simulink model "v14_registers"  (R2019b)
settings: Solver=FixedStepAuto  StartTime=0.0  StopTime=inf  FixedStep=1  MaxStep=1  RelTol=1e-3
libraries: simulink x4
settings Model: Creator=MARAT  LastModifiedBy=Marat
settings SFSimCC: CustomCodeUndefinedFunction=UseInterfaceOnly

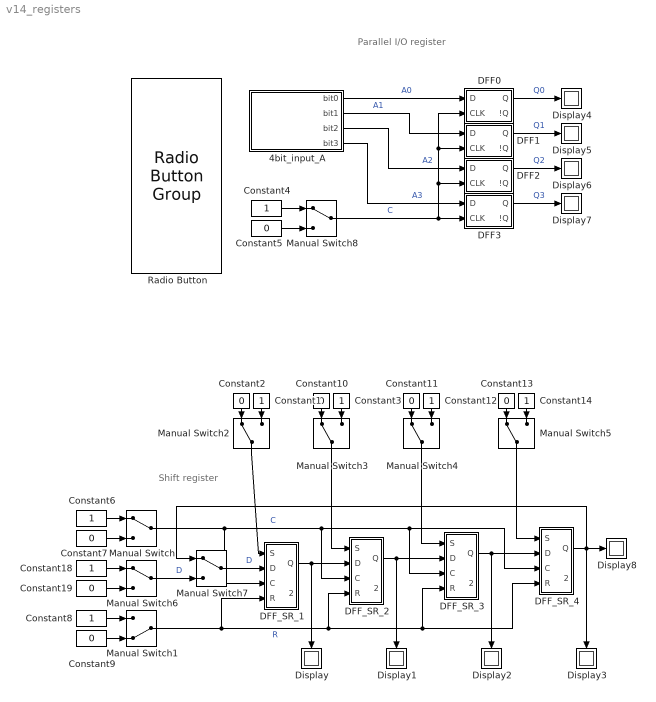
== system v14_registers ==
  note: Parallel I/O register
  note: Shift register
  4bit_input_A : Subsystem
      mask Display: image('images\sansA.png'); % Use "Edit Image" on toolstrip to change.
  Constant{1,3..4,6,8,12,14,18} (8 alike) : Constant  OutDataTypeStr=boolean
  Constant{2,5,7,9..11,13,19} (8 alike) : Constant  Value=0  OutDataTypeStr=boolean
  DFF0 : Subsystem
  DFF1 : Subsystem
  DFF2 : Subsystem
  DFF3 : Subsystem
  DFF_SR_1 : Subsystem
  DFF_SR_2 : Subsystem
  DFF_SR_3 : Subsystem
  DFF_SR_4 : Subsystem
  Display{,1..8} (9 alike) : Display
  Manual Switch{,2..8} (8 alike) : ManualSwitch
  Manual Switch1 : ManualSwitch  CurrentSetting=0
  Radio Button : RadioButtonGroup  SelectedLabel=0
      settings: Values={{'0', '1', '2', '3', '4', '5', '6', '7', '8', '9', '10', '11', '12', '13', '14', '15'}, [0 1 2 3 4 5 6 7 8 9 10 11 12 13 14 15]}
  wires:
  4bit_input_A/1(bit0) -> DFF0/1(D)  "A0"
  4bit_input_A/2(bit1) -> DFF1/1(D)  "A1"
  4bit_input_A/3(bit2) -> DFF2/1(D)  "A2"
  4bit_input_A/4(bit3) -> DFF3/1(D)  "A3"
  Constant5/1 -> Manual Switch8/2
  Constant4/1 -> Manual Switch8/1
  Manual Switch8/1 -> DFF3/2(CLK), DFF2/2(CLK), DFF1/2(CLK), DFF0/2(CLK)  "C"
  Manual Switch1/1 -> DFF_SR_4/4(R), DFF_SR_3/4(R), DFF_SR_2/4(R), DFF_SR_1/4(R)  "R"
  DFF_SR_1/1(Q) -> Display/1, DFF_SR_2/2(D)
  DFF_SR_2/1(Q) -> DFF_SR_3/2(D), Display1/1
  DFF_SR_3/1(Q) -> DFF_SR_4/2(D), Display2/1
  Constant6/1 -> Manual Switch/1
  Constant7/1 -> Manual Switch/2
  Manual Switch/1 -> DFF_SR_4/3(C), DFF_SR_3/3(C), DFF_SR_2/3(C), DFF_SR_1/3(C)  "C"
  DFF_SR_4/1(Q) -> Manual Switch7/1, Display8/1, Display3/1
  Constant9/1 -> Manual Switch1/2
  Constant8/1 -> Manual Switch1/1
  DFF0/1(Q) -> Display4/1  "Q0"
  DFF1/1(Q) -> Display5/1  "Q1"
  DFF2/1(Q) -> Display6/1  "Q2"
  DFF3/1(Q) -> Display7/1  "Q3"
  Constant19/1 -> Manual Switch6/2
  Constant18/1 -> Manual Switch6/1
  Manual Switch7/1 -> DFF_SR_1/2(D)  "D"
  Manual Switch6/1 -> Manual Switch7/2  "D"
  Manual Switch4/1 -> DFF_SR_3/1(S)
  Manual Switch5/1 -> DFF_SR_4/1(S)
  Manual Switch3/1 -> DFF_SR_2/1(S)
  Manual Switch2/1 -> DFF_SR_1/1(S)
  Constant1/1 -> Manual Switch2/2
  Constant2/1 -> Manual Switch2/1
  Constant3/1 -> Manual Switch3/2
  Constant12/1 -> Manual Switch4/2
  Constant14/1 -> Manual Switch5/2
  Constant13/1 -> Manual Switch5/1
  Constant11/1 -> Manual Switch4/1
  Constant10/1 -> Manual Switch3/1

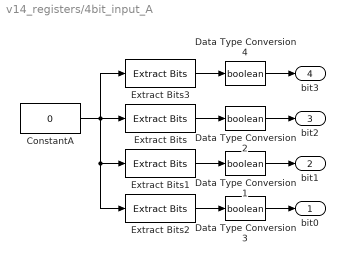
== system v14_registers/4bit_input_A ==
  ConstantA : Constant  Value=0  OutMin=0  OutMax=15  OutDataTypeStr=uint8
  Data Type Conversion{1..4} (4 alike) : DataTypeConversion  OutDataTypeStr=boolean
  Extract Bits : simulink/Logic and Bit Operations/Extract Bits  bitsToExtract=Range of bits  numBits=8  bitIdxRange=2  outScalingMode=Treat bit field as an integer
      settings: SourceProductName=Simulink
  Extract Bits1 : simulink/Logic and Bit Operations/Extract Bits  bitsToExtract=Range of bits  numBits=8  bitIdxRange=1  outScalingMode=Treat bit field as an integer
      settings: SourceProductName=Simulink
  Extract Bits2 : simulink/Logic and Bit Operations/Extract Bits  bitsToExtract=Range of bits  numBits=8  bitIdxRange=0  outScalingMode=Treat bit field as an integer
      settings: SourceProductName=Simulink
  Extract Bits3 : simulink/Logic and Bit Operations/Extract Bits  bitsToExtract=Range of bits  numBits=8  bitIdxRange=3  outScalingMode=Treat bit field as an integer
      settings: SourceProductName=Simulink
  bit0 : Outport
  bit1 : Outport  Port=2
  bit2 : Outport  Port=3
  bit3 : Outport  Port=4
  wires:
  ConstantA/1 -> Extract Bits3/1, Extract Bits2/1, Extract Bits1/1, Extract Bits/1
  Extract Bits/1 -> Data Type Conversion2/1
  Extract Bits1/1 -> Data Type Conversion1/1
  Extract Bits2/1 -> Data Type Conversion3/1
  Data Type Conversion2/1 -> bit2/1
  Data Type Conversion1/1 -> bit1/1
  Data Type Conversion3/1 -> bit0/1
  Data Type Conversion4/1 -> bit3/1
  Extract Bits3/1 -> Data Type Conversion4/1

== system v14_registers/DFF0 ==
  D : Inport
  CLK : Inport  Port=2
  Subsystem : Subsystem
  Q : Outport  InitialOutput=0  VectorParamsAs1DForOutWhenUnconnected=off
  !Q : Outport  Port=2  InitialOutput=1  VectorParamsAs1DForOutWhenUnconnected=off
  wires:
  Subsystem/2(!Q) -> !Q/1
  Subsystem/1(Q) -> Q/1
  D/1 -> Subsystem/1(D)
  CLK/1 -> Subsystem/Trigger

== system v14_registers/DFF1 ==
  D : Inport
  CLK : Inport  Port=2
  Subsystem : Subsystem
  Q : Outport  InitialOutput=0  VectorParamsAs1DForOutWhenUnconnected=off
  !Q : Outport  Port=2  InitialOutput=1  VectorParamsAs1DForOutWhenUnconnected=off
  wires:
  CLK/1 -> Subsystem/Trigger
  D/1 -> Subsystem/1(D)
  Subsystem/1(Q) -> Q/1
  Subsystem/2(!Q) -> !Q/1

== system v14_registers/DFF2 ==
  D : Inport
  CLK : Inport  Port=2
  Subsystem : Subsystem
  Q : Outport  InitialOutput=0  VectorParamsAs1DForOutWhenUnconnected=off
  !Q : Outport  Port=2  InitialOutput=1  VectorParamsAs1DForOutWhenUnconnected=off
  wires:
  Subsystem/2(!Q) -> !Q/1
  Subsystem/1(Q) -> Q/1
  D/1 -> Subsystem/1(D)
  CLK/1 -> Subsystem/Trigger

== system v14_registers/DFF3 ==
  D : Inport
  CLK : Inport  Port=2
  Subsystem : Subsystem
  Q : Outport  InitialOutput=0  VectorParamsAs1DForOutWhenUnconnected=off
  !Q : Outport  Port=2  InitialOutput=1  VectorParamsAs1DForOutWhenUnconnected=off
  wires:
  CLK/1 -> Subsystem/Trigger
  D/1 -> Subsystem/1(D)
  Subsystem/1(Q) -> Q/1
  Subsystem/2(!Q) -> !Q/1

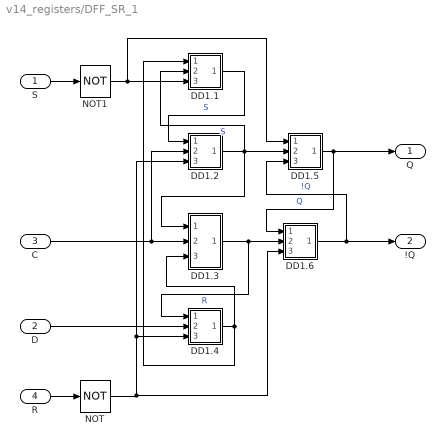
== system v14_registers/DFF_SR_1 ==
  S : Inport
  D : Inport  Port=2
  C : Inport  Port=3
  R : Inport  Port=4
  DD1.1 : Subsystem
      mask Display: disp('&~');
  DD1.2 : Subsystem
      mask Display: disp('&~');
  DD1.3 : Subsystem
      mask Display: disp('&~');
  DD1.4 : Subsystem
      mask Display: disp('&~');
  DD1.5 : Subsystem
      mask Display: disp('&~');
  DD1.6 : Subsystem
      mask Display: disp('&~');
  NOT : Logic  Operator=NOT  IconShape=distinctive  AllPortsSameDT=off  OutDataTypeStr=boolean
  NOT1 : Logic  Operator=NOT  IconShape=distinctive  AllPortsSameDT=off  OutDataTypeStr=boolean
  Q : Outport
  !Q : Outport  Port=2
  wires:
  DD1.5/1(Out1) -> Q/1, DD1.6/1(In1)  "Q"
  R/1 -> NOT/1
  DD1.4/1(Out1) -> DD1.1/1(In1), DD1.3/3(In3)
  C/1 -> DD1.2/2(In2), DD1.3/2(In2)
  S/1 -> NOT1/1
  DD1.3/1(Out1) -> DD1.6/2(In2), DD1.4/1(In1)  "R"
  DD1.1/1(Out1) -> DD1.2/1(In1)  "S"
  DD1.6/1(Out1) -> !Q/1, DD1.5/3(In3)  "!Q"
  D/1 -> DD1.4/2(In2)
  DD1.2/1(Out1) -> DD1.3/1(In1), DD1.5/2(In2), DD1.1/2(In2)  "S"
  NOT/1 -> DD1.6/3(In3), DD1.4/3(In3), DD1.2/3(In3)
  NOT1/1 -> DD1.5/1(In1), DD1.1/3(In3)

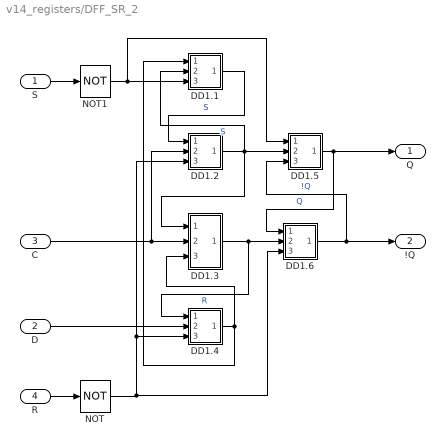
== system v14_registers/DFF_SR_2 ==
  S : Inport
  D : Inport  Port=2
  C : Inport  Port=3
  R : Inport  Port=4
  DD1.1 : Subsystem
      mask Display: disp('&~');
  DD1.2 : Subsystem
      mask Display: disp('&~');
  DD1.3 : Subsystem
      mask Display: disp('&~');
  DD1.4 : Subsystem
      mask Display: disp('&~');
  DD1.5 : Subsystem
      mask Display: disp('&~');
  DD1.6 : Subsystem
      mask Display: disp('&~');
  NOT : Logic  Operator=NOT  IconShape=distinctive  AllPortsSameDT=off  OutDataTypeStr=boolean
  NOT1 : Logic  Operator=NOT  IconShape=distinctive  AllPortsSameDT=off  OutDataTypeStr=boolean
  Q : Outport
  !Q : Outport  Port=2
  wires:
  NOT1/1 -> DD1.1/3(In3), DD1.5/1(In1)
  NOT/1 -> DD1.2/3(In3), DD1.4/3(In3), DD1.6/3(In3)
  DD1.2/1(Out1) -> DD1.1/2(In2), DD1.5/2(In2), DD1.3/1(In1)  "S"
  D/1 -> DD1.4/2(In2)
  DD1.6/1(Out1) -> DD1.5/3(In3), !Q/1  "!Q"
  DD1.1/1(Out1) -> DD1.2/1(In1)  "S"
  DD1.3/1(Out1) -> DD1.4/1(In1), DD1.6/2(In2)  "R"
  S/1 -> NOT1/1
  C/1 -> DD1.3/2(In2), DD1.2/2(In2)
  DD1.4/1(Out1) -> DD1.3/3(In3), DD1.1/1(In1)
  R/1 -> NOT/1
  DD1.5/1(Out1) -> DD1.6/1(In1), Q/1  "Q"

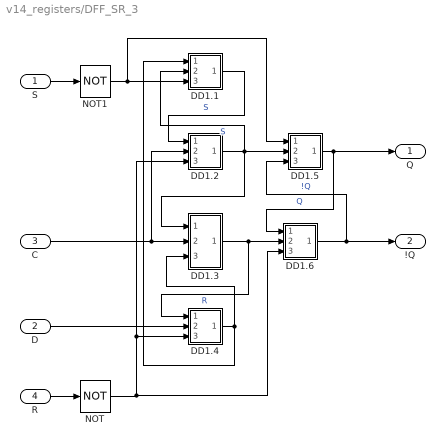
== system v14_registers/DFF_SR_3 ==
  S : Inport
  D : Inport  Port=2
  C : Inport  Port=3
  R : Inport  Port=4
  DD1.1 : Subsystem
      mask Display: disp('&~');
  DD1.2 : Subsystem
      mask Display: disp('&~');
  DD1.3 : Subsystem
      mask Display: disp('&~');
  DD1.4 : Subsystem
      mask Display: disp('&~');
  DD1.5 : Subsystem
      mask Display: disp('&~');
  DD1.6 : Subsystem
      mask Display: disp('&~');
  NOT : Logic  Operator=NOT  IconShape=distinctive  AllPortsSameDT=off  OutDataTypeStr=boolean
  NOT1 : Logic  Operator=NOT  IconShape=distinctive  AllPortsSameDT=off  OutDataTypeStr=boolean
  Q : Outport
  !Q : Outport  Port=2
  wires:
  NOT1/1 -> DD1.1/3(In3), DD1.5/1(In1)
  NOT/1 -> DD1.2/3(In3), DD1.4/3(In3), DD1.6/3(In3)
  DD1.2/1(Out1) -> DD1.1/2(In2), DD1.5/2(In2), DD1.3/1(In1)  "S"
  D/1 -> DD1.4/2(In2)
  DD1.6/1(Out1) -> DD1.5/3(In3), !Q/1  "!Q"
  DD1.1/1(Out1) -> DD1.2/1(In1)  "S"
  DD1.3/1(Out1) -> DD1.4/1(In1), DD1.6/2(In2)  "R"
  S/1 -> NOT1/1
  C/1 -> DD1.3/2(In2), DD1.2/2(In2)
  DD1.4/1(Out1) -> DD1.3/3(In3), DD1.1/1(In1)
  R/1 -> NOT/1
  DD1.5/1(Out1) -> DD1.6/1(In1), Q/1  "Q"

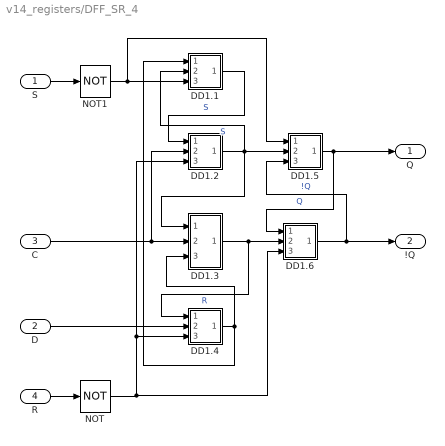
== system v14_registers/DFF_SR_4 ==
  S : Inport
  D : Inport  Port=2
  C : Inport  Port=3
  R : Inport  Port=4
  DD1.1 : Subsystem
      mask Display: disp('&~');
  DD1.2 : Subsystem
      mask Display: disp('&~');
  DD1.3 : Subsystem
      mask Display: disp('&~');
  DD1.4 : Subsystem
      mask Display: disp('&~');
  DD1.5 : Subsystem
      mask Display: disp('&~');
  DD1.6 : Subsystem
      mask Display: disp('&~');
  NOT : Logic  Operator=NOT  IconShape=distinctive  AllPortsSameDT=off  OutDataTypeStr=boolean
  NOT1 : Logic  Operator=NOT  IconShape=distinctive  AllPortsSameDT=off  OutDataTypeStr=boolean
  Q : Outport
  !Q : Outport  Port=2
  wires:
  DD1.5/1(Out1) -> Q/1, DD1.6/1(In1)  "Q"
  R/1 -> NOT/1
  DD1.4/1(Out1) -> DD1.1/1(In1), DD1.3/3(In3)
  C/1 -> DD1.2/2(In2), DD1.3/2(In2)
  S/1 -> NOT1/1
  DD1.3/1(Out1) -> DD1.6/2(In2), DD1.4/1(In1)  "R"
  DD1.1/1(Out1) -> DD1.2/1(In1)  "S"
  DD1.6/1(Out1) -> !Q/1, DD1.5/3(In3)  "!Q"
  D/1 -> DD1.4/2(In2)
  DD1.2/1(Out1) -> DD1.3/1(In1), DD1.5/2(In2), DD1.1/2(In2)  "S"
  NOT/1 -> DD1.6/3(In3), DD1.4/3(In3), DD1.2/3(In3)
  NOT1/1 -> DD1.5/1(In1), DD1.1/3(In3)

== system v14_registers/DFF0/Subsystem ==
  D : Inport  LatchByDelayingOutsideSignal=on
  Trigger : TriggerPort  VariantControl=Variant  StatesWhenEnabling=reset
  Logic : Logic  Operator=NOT  Inputs=1
  Q : Outport  OutputWhenDisabled=reset  InitialOutput=0  VectorParamsAs1DForOutWhenUnconnected=off
  !Q : Outport  Port=2  OutputWhenDisabled=reset  InitialOutput=1  VectorParamsAs1DForOutWhenUnconnected=off
  wires:
  D/1 -> Logic/1, Q/1
  Logic/1 -> !Q/1

== system v14_registers/DFF1/Subsystem ==
  D : Inport  LatchByDelayingOutsideSignal=on
  Trigger : TriggerPort  VariantControl=Variant  StatesWhenEnabling=reset
  Logic : Logic  Operator=NOT  Inputs=1
  Q : Outport  OutputWhenDisabled=reset  InitialOutput=0  VectorParamsAs1DForOutWhenUnconnected=off
  !Q : Outport  Port=2  OutputWhenDisabled=reset  InitialOutput=1  VectorParamsAs1DForOutWhenUnconnected=off
  wires:
  Logic/1 -> !Q/1
  D/1 -> Q/1, Logic/1

== system v14_registers/DFF2/Subsystem ==
  D : Inport  LatchByDelayingOutsideSignal=on
  Trigger : TriggerPort  VariantControl=Variant  StatesWhenEnabling=reset
  Logic : Logic  Operator=NOT  Inputs=1
  Q : Outport  OutputWhenDisabled=reset  InitialOutput=0  VectorParamsAs1DForOutWhenUnconnected=off
  !Q : Outport  Port=2  OutputWhenDisabled=reset  InitialOutput=1  VectorParamsAs1DForOutWhenUnconnected=off
  wires:
  D/1 -> Logic/1, Q/1
  Logic/1 -> !Q/1

== system v14_registers/DFF3/Subsystem ==
  D : Inport  LatchByDelayingOutsideSignal=on
  Trigger : TriggerPort  VariantControl=Variant  StatesWhenEnabling=reset
  Logic : Logic  Operator=NOT  Inputs=1
  Q : Outport  OutputWhenDisabled=reset  InitialOutput=0  VectorParamsAs1DForOutWhenUnconnected=off
  !Q : Outport  Port=2  OutputWhenDisabled=reset  InitialOutput=1  VectorParamsAs1DForOutWhenUnconnected=off
  wires:
  Logic/1 -> !Q/1
  D/1 -> Q/1, Logic/1

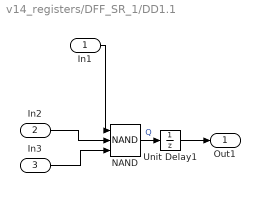
== system v14_registers/DFF_SR_1/DD1.1 ==
  In1 : Inport
  In2 : Inport  Port=2
  In3 : Inport  Port=3
  NAND : Logic  Operator=NAND  Inputs=3  IconShape=distinctive  AllPortsSameDT=off  OutDataTypeStr=boolean
  Unit Delay1 : UnitDelay  SampleTime=-1  HasFrameUpgradeWarning=on
  Out1 : Outport
  wires:
  In2/1 -> NAND/2
  In1/1 -> NAND/1
  Unit Delay1/1 -> Out1/1
  NAND/1 -> Unit Delay1/1  "Q"
  In3/1 -> NAND/3

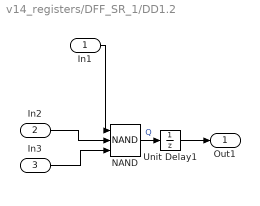
== system v14_registers/DFF_SR_1/DD1.2 ==
  In1 : Inport
  In2 : Inport  Port=2
  In3 : Inport  Port=3
  NAND : Logic  Operator=NAND  Inputs=3  IconShape=distinctive  AllPortsSameDT=off  OutDataTypeStr=boolean
  Unit Delay1 : UnitDelay  SampleTime=-1  HasFrameUpgradeWarning=on
  Out1 : Outport
  wires:
  In3/1 -> NAND/3
  NAND/1 -> Unit Delay1/1  "Q"
  Unit Delay1/1 -> Out1/1
  In1/1 -> NAND/1
  In2/1 -> NAND/2

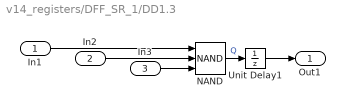
== system v14_registers/DFF_SR_1/DD1.3 ==
  In1 : Inport
  In2 : Inport  Port=2
  In3 : Inport  Port=3
  NAND : Logic  Operator=NAND  Inputs=3  IconShape=distinctive  AllPortsSameDT=off  OutDataTypeStr=boolean
  Unit Delay1 : UnitDelay  SampleTime=-1  HasFrameUpgradeWarning=on
  Out1 : Outport
  wires:
  In3/1 -> NAND/3
  In2/1 -> NAND/2
  In1/1 -> NAND/1
  Unit Delay1/1 -> Out1/1
  NAND/1 -> Unit Delay1/1  "Q"

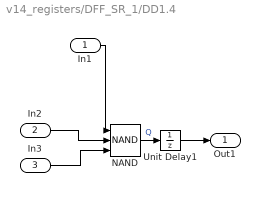
== system v14_registers/DFF_SR_1/DD1.4 ==
  In1 : Inport
  In2 : Inport  Port=2
  In3 : Inport  Port=3
  NAND : Logic  Operator=NAND  Inputs=3  IconShape=distinctive  AllPortsSameDT=off  OutDataTypeStr=boolean
  Unit Delay1 : UnitDelay  SampleTime=-1  HasFrameUpgradeWarning=on
  Out1 : Outport
  wires:
  In2/1 -> NAND/2
  In1/1 -> NAND/1
  Unit Delay1/1 -> Out1/1
  NAND/1 -> Unit Delay1/1  "Q"
  In3/1 -> NAND/3

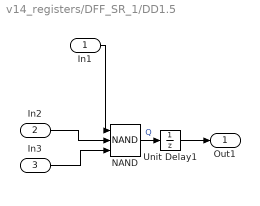
== system v14_registers/DFF_SR_1/DD1.5 ==
  In1 : Inport
  In2 : Inport  Port=2
  In3 : Inport  Port=3
  NAND : Logic  Operator=NAND  Inputs=3  IconShape=distinctive  AllPortsSameDT=off  OutDataTypeStr=boolean
  Unit Delay1 : UnitDelay  SampleTime=-1  HasFrameUpgradeWarning=on
  Out1 : Outport
  wires:
  In3/1 -> NAND/3
  NAND/1 -> Unit Delay1/1  "Q"
  Unit Delay1/1 -> Out1/1
  In1/1 -> NAND/1
  In2/1 -> NAND/2

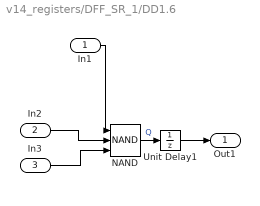
== system v14_registers/DFF_SR_1/DD1.6 ==
  In1 : Inport
  In2 : Inport  Port=2
  In3 : Inport  Port=3
  NAND : Logic  Operator=NAND  Inputs=3  IconShape=distinctive  AllPortsSameDT=off  OutDataTypeStr=boolean
  Unit Delay1 : UnitDelay  SampleTime=-1  HasFrameUpgradeWarning=on
  Out1 : Outport
  wires:
  In2/1 -> NAND/2
  In1/1 -> NAND/1
  Unit Delay1/1 -> Out1/1
  NAND/1 -> Unit Delay1/1  "Q"
  In3/1 -> NAND/3

== system v14_registers/DFF_SR_2/DD1.1 ==
  In1 : Inport
  In2 : Inport  Port=2
  In3 : Inport  Port=3
  NAND : Logic  Operator=NAND  Inputs=3  IconShape=distinctive  AllPortsSameDT=off  OutDataTypeStr=boolean
  Unit Delay1 : UnitDelay  SampleTime=-1  HasFrameUpgradeWarning=on
  Out1 : Outport
  wires:
  In3/1 -> NAND/3
  NAND/1 -> Unit Delay1/1  "Q"
  Unit Delay1/1 -> Out1/1
  In1/1 -> NAND/1
  In2/1 -> NAND/2

== system v14_registers/DFF_SR_2/DD1.2 ==
  In1 : Inport
  In2 : Inport  Port=2
  In3 : Inport  Port=3
  NAND : Logic  Operator=NAND  Inputs=3  IconShape=distinctive  AllPortsSameDT=off  OutDataTypeStr=boolean
  Unit Delay1 : UnitDelay  SampleTime=-1  HasFrameUpgradeWarning=on
  Out1 : Outport
  wires:
  In2/1 -> NAND/2
  In1/1 -> NAND/1
  Unit Delay1/1 -> Out1/1
  NAND/1 -> Unit Delay1/1  "Q"
  In3/1 -> NAND/3

== system v14_registers/DFF_SR_2/DD1.3 ==
  In1 : Inport
  In2 : Inport  Port=2
  In3 : Inport  Port=3
  NAND : Logic  Operator=NAND  Inputs=3  IconShape=distinctive  AllPortsSameDT=off  OutDataTypeStr=boolean
  Unit Delay1 : UnitDelay  SampleTime=-1  HasFrameUpgradeWarning=on
  Out1 : Outport
  wires:
  NAND/1 -> Unit Delay1/1  "Q"
  Unit Delay1/1 -> Out1/1
  In1/1 -> NAND/1
  In2/1 -> NAND/2
  In3/1 -> NAND/3

== system v14_registers/DFF_SR_2/DD1.4 ==
  In1 : Inport
  In2 : Inport  Port=2
  In3 : Inport  Port=3
  NAND : Logic  Operator=NAND  Inputs=3  IconShape=distinctive  AllPortsSameDT=off  OutDataTypeStr=boolean
  Unit Delay1 : UnitDelay  SampleTime=-1  HasFrameUpgradeWarning=on
  Out1 : Outport
  wires:
  In3/1 -> NAND/3
  NAND/1 -> Unit Delay1/1  "Q"
  Unit Delay1/1 -> Out1/1
  In1/1 -> NAND/1
  In2/1 -> NAND/2

== system v14_registers/DFF_SR_2/DD1.5 ==
  In1 : Inport
  In2 : Inport  Port=2
  In3 : Inport  Port=3
  NAND : Logic  Operator=NAND  Inputs=3  IconShape=distinctive  AllPortsSameDT=off  OutDataTypeStr=boolean
  Unit Delay1 : UnitDelay  SampleTime=-1  HasFrameUpgradeWarning=on
  Out1 : Outport
  wires:
  In2/1 -> NAND/2
  In1/1 -> NAND/1
  Unit Delay1/1 -> Out1/1
  NAND/1 -> Unit Delay1/1  "Q"
  In3/1 -> NAND/3

== system v14_registers/DFF_SR_2/DD1.6 ==
  In1 : Inport
  In2 : Inport  Port=2
  In3 : Inport  Port=3
  NAND : Logic  Operator=NAND  Inputs=3  IconShape=distinctive  AllPortsSameDT=off  OutDataTypeStr=boolean
  Unit Delay1 : UnitDelay  SampleTime=-1  HasFrameUpgradeWarning=on
  Out1 : Outport
  wires:
  In3/1 -> NAND/3
  NAND/1 -> Unit Delay1/1  "Q"
  Unit Delay1/1 -> Out1/1
  In1/1 -> NAND/1
  In2/1 -> NAND/2

== system v14_registers/DFF_SR_3/DD1.1 ==
  In1 : Inport
  In2 : Inport  Port=2
  In3 : Inport  Port=3
  NAND : Logic  Operator=NAND  Inputs=3  IconShape=distinctive  AllPortsSameDT=off  OutDataTypeStr=boolean
  Unit Delay1 : UnitDelay  SampleTime=-1  HasFrameUpgradeWarning=on
  Out1 : Outport
  wires:
  In3/1 -> NAND/3
  NAND/1 -> Unit Delay1/1  "Q"
  Unit Delay1/1 -> Out1/1
  In1/1 -> NAND/1
  In2/1 -> NAND/2

== system v14_registers/DFF_SR_3/DD1.2 ==
  In1 : Inport
  In2 : Inport  Port=2
  In3 : Inport  Port=3
  NAND : Logic  Operator=NAND  Inputs=3  IconShape=distinctive  AllPortsSameDT=off  OutDataTypeStr=boolean
  Unit Delay1 : UnitDelay  SampleTime=-1  HasFrameUpgradeWarning=on
  Out1 : Outport
  wires:
  In2/1 -> NAND/2
  In1/1 -> NAND/1
  Unit Delay1/1 -> Out1/1
  NAND/1 -> Unit Delay1/1  "Q"
  In3/1 -> NAND/3

== system v14_registers/DFF_SR_3/DD1.3 ==
  In1 : Inport
  In2 : Inport  Port=2
  In3 : Inport  Port=3
  NAND : Logic  Operator=NAND  Inputs=3  IconShape=distinctive  AllPortsSameDT=off  OutDataTypeStr=boolean
  Unit Delay1 : UnitDelay  SampleTime=-1  HasFrameUpgradeWarning=on
  Out1 : Outport
  wires:
  NAND/1 -> Unit Delay1/1  "Q"
  Unit Delay1/1 -> Out1/1
  In1/1 -> NAND/1
  In2/1 -> NAND/2
  In3/1 -> NAND/3

== system v14_registers/DFF_SR_3/DD1.4 ==
  In1 : Inport
  In2 : Inport  Port=2
  In3 : Inport  Port=3
  NAND : Logic  Operator=NAND  Inputs=3  IconShape=distinctive  AllPortsSameDT=off  OutDataTypeStr=boolean
  Unit Delay1 : UnitDelay  SampleTime=-1  HasFrameUpgradeWarning=on
  Out1 : Outport
  wires:
  In3/1 -> NAND/3
  NAND/1 -> Unit Delay1/1  "Q"
  Unit Delay1/1 -> Out1/1
  In1/1 -> NAND/1
  In2/1 -> NAND/2

== system v14_registers/DFF_SR_3/DD1.5 ==
  In1 : Inport
  In2 : Inport  Port=2
  In3 : Inport  Port=3
  NAND : Logic  Operator=NAND  Inputs=3  IconShape=distinctive  AllPortsSameDT=off  OutDataTypeStr=boolean
  Unit Delay1 : UnitDelay  SampleTime=-1  HasFrameUpgradeWarning=on
  Out1 : Outport
  wires:
  In2/1 -> NAND/2
  In1/1 -> NAND/1
  Unit Delay1/1 -> Out1/1
  NAND/1 -> Unit Delay1/1  "Q"
  In3/1 -> NAND/3

== system v14_registers/DFF_SR_3/DD1.6 ==
  In1 : Inport
  In2 : Inport  Port=2
  In3 : Inport  Port=3
  NAND : Logic  Operator=NAND  Inputs=3  IconShape=distinctive  AllPortsSameDT=off  OutDataTypeStr=boolean
  Unit Delay1 : UnitDelay  SampleTime=-1  HasFrameUpgradeWarning=on
  Out1 : Outport
  wires:
  In3/1 -> NAND/3
  NAND/1 -> Unit Delay1/1  "Q"
  Unit Delay1/1 -> Out1/1
  In1/1 -> NAND/1
  In2/1 -> NAND/2

== system v14_registers/DFF_SR_4/DD1.1 ==
  In1 : Inport
  In2 : Inport  Port=2
  In3 : Inport  Port=3
  NAND : Logic  Operator=NAND  Inputs=3  IconShape=distinctive  AllPortsSameDT=off  OutDataTypeStr=boolean
  Unit Delay1 : UnitDelay  SampleTime=-1  HasFrameUpgradeWarning=on
  Out1 : Outport
  wires:
  In2/1 -> NAND/2
  In1/1 -> NAND/1
  Unit Delay1/1 -> Out1/1
  NAND/1 -> Unit Delay1/1  "Q"
  In3/1 -> NAND/3

== system v14_registers/DFF_SR_4/DD1.2 ==
  In1 : Inport
  In2 : Inport  Port=2
  In3 : Inport  Port=3
  NAND : Logic  Operator=NAND  Inputs=3  IconShape=distinctive  AllPortsSameDT=off  OutDataTypeStr=boolean
  Unit Delay1 : UnitDelay  SampleTime=-1  HasFrameUpgradeWarning=on
  Out1 : Outport
  wires:
  In3/1 -> NAND/3
  NAND/1 -> Unit Delay1/1  "Q"
  Unit Delay1/1 -> Out1/1
  In1/1 -> NAND/1
  In2/1 -> NAND/2

== system v14_registers/DFF_SR_4/DD1.3 ==
  In1 : Inport
  In2 : Inport  Port=2
  In3 : Inport  Port=3
  NAND : Logic  Operator=NAND  Inputs=3  IconShape=distinctive  AllPortsSameDT=off  OutDataTypeStr=boolean
  Unit Delay1 : UnitDelay  SampleTime=-1  HasFrameUpgradeWarning=on
  Out1 : Outport
  wires:
  In3/1 -> NAND/3
  In2/1 -> NAND/2
  In1/1 -> NAND/1
  Unit Delay1/1 -> Out1/1
  NAND/1 -> Unit Delay1/1  "Q"

== system v14_registers/DFF_SR_4/DD1.4 ==
  In1 : Inport
  In2 : Inport  Port=2
  In3 : Inport  Port=3
  NAND : Logic  Operator=NAND  Inputs=3  IconShape=distinctive  AllPortsSameDT=off  OutDataTypeStr=boolean
  Unit Delay1 : UnitDelay  SampleTime=-1  HasFrameUpgradeWarning=on
  Out1 : Outport
  wires:
  In2/1 -> NAND/2
  In1/1 -> NAND/1
  Unit Delay1/1 -> Out1/1
  NAND/1 -> Unit Delay1/1  "Q"
  In3/1 -> NAND/3

== system v14_registers/DFF_SR_4/DD1.5 ==
  In1 : Inport
  In2 : Inport  Port=2
  In3 : Inport  Port=3
  NAND : Logic  Operator=NAND  Inputs=3  IconShape=distinctive  AllPortsSameDT=off  OutDataTypeStr=boolean
  Unit Delay1 : UnitDelay  SampleTime=-1  HasFrameUpgradeWarning=on
  Out1 : Outport
  wires:
  In3/1 -> NAND/3
  NAND/1 -> Unit Delay1/1  "Q"
  Unit Delay1/1 -> Out1/1
  In1/1 -> NAND/1
  In2/1 -> NAND/2

== system v14_registers/DFF_SR_4/DD1.6 ==
  In1 : Inport
  In2 : Inport  Port=2
  In3 : Inport  Port=3
  NAND : Logic  Operator=NAND  Inputs=3  IconShape=distinctive  AllPortsSameDT=off  OutDataTypeStr=boolean
  Unit Delay1 : UnitDelay  SampleTime=-1  HasFrameUpgradeWarning=on
  Out1 : Outport
  wires:
  In2/1 -> NAND/2
  In1/1 -> NAND/1
  Unit Delay1/1 -> Out1/1
  NAND/1 -> Unit Delay1/1  "Q"
  In3/1 -> NAND/3
